simulink model "C4_closedLoopPositionPD"  (Simulink 10.2)
settings: Solver=ode4  StartTime=0.0  StopTime=1  FixedStep=T_s  RelTol=1e-3
undefined symbols (not defined in the file): b_eq, beta_p, beta_v, g, i_rated, J_eq, k, k_d_pos, k_p_currPI, k_p_pos, L, L_l, m_l, N_adc, N_e, N_opt, R, R_sh, T_i_currPI, T_s, tau_der, tau_m_rated, theta_0, theta_ref, V_adc
libraries: simulink x1
settings Model: Creator=ioannis  LastModifiedBy=mfocchi
settings DataIOCC: SaveFormat=Dataset  SignalLoggingSaveFormat=Dataset
settings OptimizationCC: LifeSpan=auto
settings DebuggingCC: UnderspecifiedInitializationDetection=Simplified  MergeDetectMultiDrivingBlocksExec=error  FcnCallInpInsideContextMsg=error  SFUnexpectedBacktrackingDiag=error  SFNoUnconditionalDefaultTransitionDiag=error  SFExecutionAtInitializationDiag=warning
settings HardwareCC: ProdBitPerPointer=64  ProdBitPerSizeT=64  ProdBitPerPtrDiffT=64  ProdLargestAtomicFloat=Float  ProdIntDivRoundTo=Zero  ProdEndianess=LittleEndian  ProdWordSize=64  ProdHWDeviceType=Intel->x86-64 (Windows64)
settings ModelReferenceCC: PropagateSignalLabelsOutOfModel=on
settings SFSimCC: SimUseLocalCustomCode=on
settings RTWCC: RTWUseLocalCustomCode=on
settings CodeAppCC: StateflowObjectComments=off
settings GRTTargetCC: TargetLangStandard=C99 (ISO)  CombineOutputUpdateFcns=on  GRTInterface=off
settings ConfigComp: CovMetricSettings=dwe  CovSaveCumulativeToWorkspaceVar=off  CovSaveSingleToWorkspaceVar=off  CovExternalEMLEnable=on

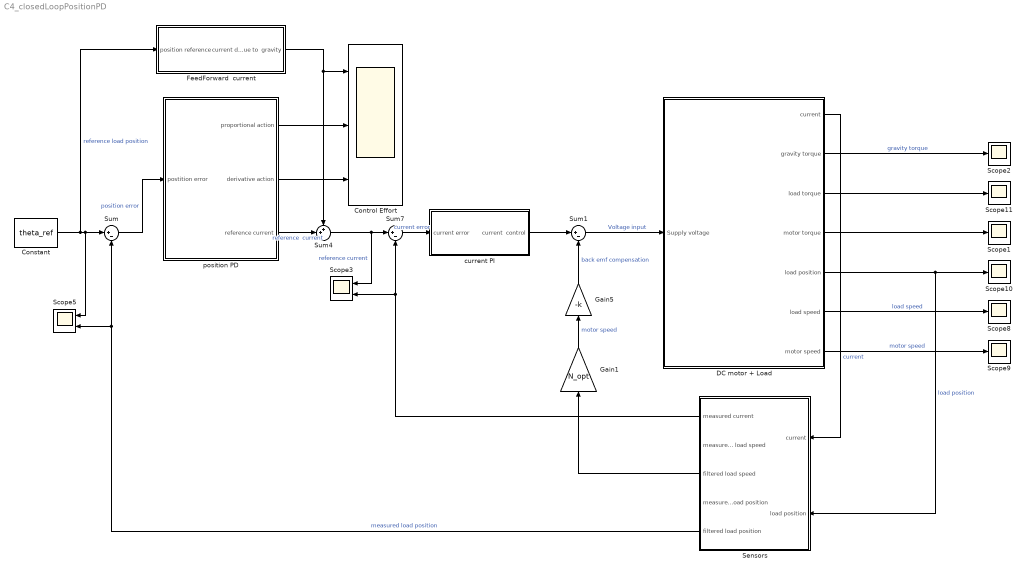
== system C4_closedLoopPositionPD ==
  Constant : Constant  Value=theta_ref
  Control Effort : Scope  NumInputPorts=3
  DC motor + Load : Subsystem
  FeedForward  current : Subsystem
  Gain1 : Gain  Gain=N_opt
  Gain5 : Gain  Gain=-k
  Scope{1..2,8..11} (6 alike) : Scope
  Scope3 : Scope  NumInputPorts=2
  Scope5 : Scope  NumInputPorts=2
  Sensors : Subsystem
  Sum : Sum  Inputs=|+-
  Sum1 : Sum  Inputs=|+-
  Sum4 : Sum  Inputs=++|
  Sum7 : Sum  Inputs=|+-
  current PI : Subsystem
  position PD : Subsystem
  wires:
  Sum7/1 -> current PI/1(current error)  "current error"
  Sum1/1 -> DC motor + Load/1(Supply voltage)  "Voltage input"
  DC motor + Load/4(motor torque) -> Scope1/1
  DC motor + Load/5(load position) -> Sensors/2(load position), Scope10/1  "load position"
  DC motor + Load/6(load speed) -> Scope8/1  "load speed"
  DC motor + Load/7(motor speed) -> Scope9/1  "motor speed"
  DC motor + Load/2(gravity torque) -> Scope2/1  "gravity torque"
  DC motor + Load/3(load torque) -> Scope11/1
  Gain1/1 -> Gain5/1  "motor speed"
  DC motor + Load/1(current) -> Sensors/1(current)  "current"
  Sensors/3(filtered load speed) -> Gain1/1
  Gain5/1 -> Sum1/2  "back emf compensation"
  Sensors/1(measured current) -> Scope3/2, Sum7/2
  Sum/1 -> position PD/1(postition error)  "position error"
  Sensors/5(filtered load position) -> Scope5/2, Sum/2  "measured load position"
  Constant/1 -> FeedForward  current/1(position reference), Scope5/1, Sum/1  "reference load position"
  current PI/1(current  control) -> Sum1/1
  Sum4/1 -> Scope3/1, Sum7/1  "reference current"
  position PD/3(reference current) -> Sum4/2  "reference  current"
  position PD/2(derivative action) -> Control Effort/3
  position PD/1(proportional action) -> Control Effort/2
  FeedForward  current/1(current due to  gravity) -> Sum4/1, Control Effort/1

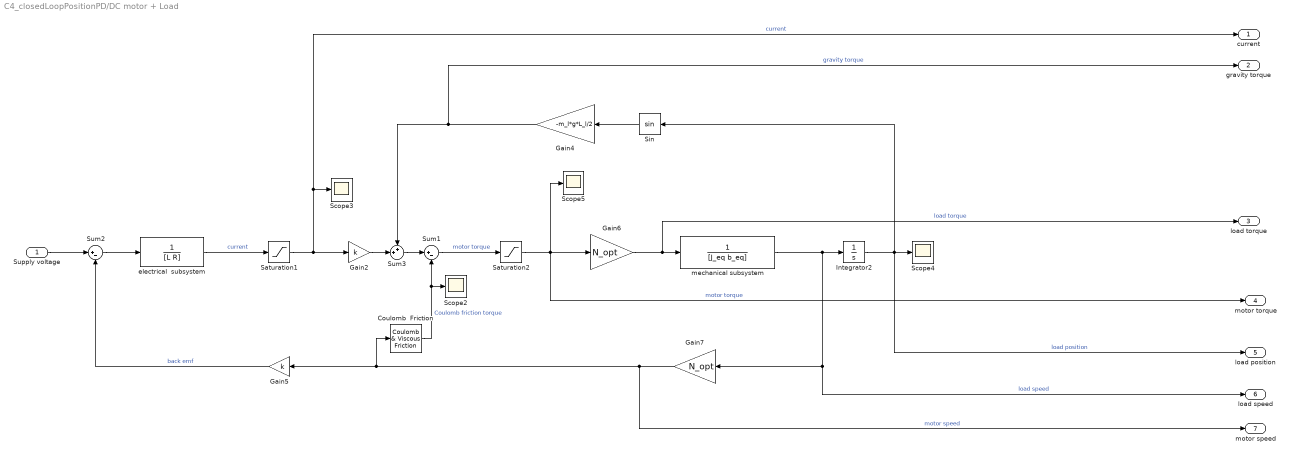
== system C4_closedLoopPositionPD/DC motor + Load ==
  Supply voltage : Inport
  Coulomb  Friction : simulink/Discontinuities/Coulomb & Viscous Friction  offset=tau_c  gain=0
  Gain2 : Gain  Gain=k
  Gain4 : Gain  Gain=-m_l*g*L_l/2
  Gain5 : Gain  Gain=k
  Gain6 : Gain  Gain=N_opt
  Gain7 : Gain  Gain=N_opt
  Integrator2 : Integrator  InitialCondition=theta_0
  Saturation1 : Saturate  UpperLimit=i_rated  LowerLimit=-i_rated
  Saturation2 : Saturate  UpperLimit=tau_m_rated  LowerLimit=-tau_m_rated
  Scope{2..5} (4 alike) : Scope
  Sin : Trigonometry
  Sum1 : Sum  Inputs=|+-
  Sum2 : Sum  Inputs=|+-
  Sum3 : Sum  Inputs=++|
  electrical  subsystem : TransferFcn  Denominator=[L R]
  mechanical subsystem : TransferFcn  Denominator=[J_eq b_eq]
  current : Outport
  gravity torque : Outport  Port=2
  load torque : Outport  Port=3
  motor torque : Outport  Port=4
  load position : Outport  Port=5
  load speed : Outport  Port=6
  motor speed : Outport  Port=7
  wires:
  Sum2/1 -> electrical  subsystem/1
  Saturation2/1 -> motor torque/1, Scope5/1, Gain6/1  "motor torque"
  Sum3/1 -> Sum1/1
  Sum1/1 -> Saturation2/1  "motor torque"
  Sin/1 -> Gain4/1
  Gain5/1 -> Sum2/2  "back emf"
  electrical  subsystem/1 -> Saturation1/1  "current"
  Gain2/1 -> Sum3/2
  Gain6/1 -> load torque/1, mechanical subsystem/1  "load torque"
  mechanical subsystem/1 -> Gain7/1, load speed/1, Integrator2/1  "load speed"
  Supply voltage/1 -> Sum2/1
  Integrator2/1 -> Sin/1, load position/1, Scope4/1  "load position"
  Gain4/1 -> gravity torque/1, Sum3/1  "gravity torque"
  Saturation1/1 -> current/1, Scope3/1, Gain2/1  "current"
  Gain7/1 -> motor speed/1, Coulomb  Friction/1, Gain5/1  "motor speed"
  Coulomb  Friction/1 -> Sum1/2, Scope2/1  "Coulomb friction torque"

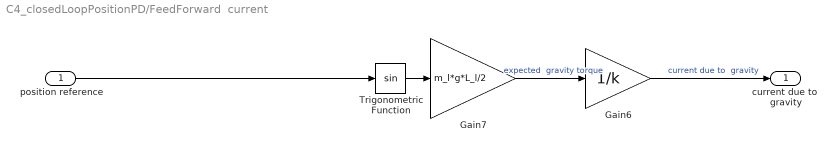
== system C4_closedLoopPositionPD/FeedForward  current ==
  position reference : Inport
  Gain6 : Gain  Gain=1/k
  Gain7 : Gain  Gain=m_l*g*L_l/2
  Trigonometric Function : Trigonometry
  current due to  gravity : Outport
  wires:
  position reference/1 -> Trigonometric Function/1
  Gain6/1 -> current due to  gravity/1  "current due to  gravity"
  Gain7/1 -> Gain6/1  "expected  gravity torque"
  Trigonometric Function/1 -> Gain7/1

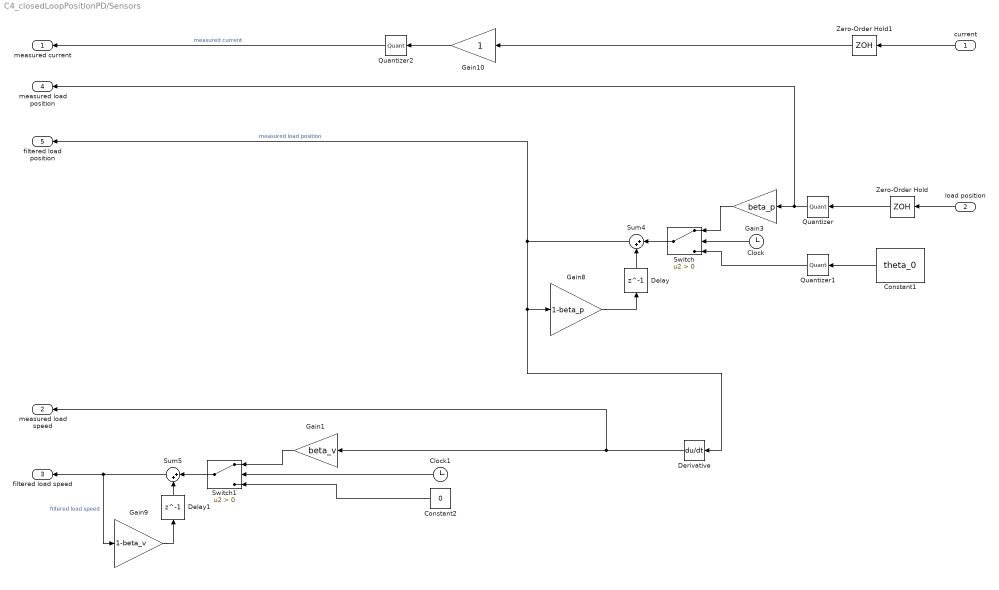
== system C4_closedLoopPositionPD/Sensors ==
  current : Inport
  load position : Inport  Port=2
  Clock : Clock
  Clock1 : Clock
  Constant1 : Constant  Value=theta_0
  Constant2 : Constant  Value=0
  Delay : Delay  DelayLength=1  InitialCondition=0
  Delay1 : Delay  DelayLength=1  InitialCondition=0
  Derivative : Derivative
  Gain1 : Gain  Gain=beta_v
  Gain10 : Gain
  Gain3 : Gain  Gain=beta_p
  Gain8 : Gain  Gain=1-beta_p
  Gain9 : Gain  Gain=1-beta_v
  Quantizer : Quantizer  QuantizationInterval=2*pi/(2^N_e)
  Quantizer1 : Quantizer  QuantizationInterval=2*pi/(2^N_e)
  Quantizer2 : Quantizer  QuantizationInterval=V_adc/R_sh/(2^N_adc)
  Sum4 : Sum  Inputs=|++
  Sum5 : Sum  Inputs=|++
  Switch : Switch  Criteria=u2 > Threshold
  Switch1 : Switch  Criteria=u2 > Threshold
  Zero-Order Hold : ZeroOrderHold  SampleTime=T_s
  Zero-Order Hold1 : ZeroOrderHold  SampleTime=T_s
  measured current : Outport
  measured load speed : Outport  Port=2
  filtered load speed : Outport  Port=3
  measured load position : Outport  Port=4
  filtered load position : Outport  Port=5
  wires:
  Gain3/1 -> Switch/1
  Switch/1 -> Sum4/1
  Quantizer/1 -> measured load position/1, Gain3/1
  Constant1/1 -> Quantizer1/1
  Delay/1 -> Sum4/2
  Quantizer1/1 -> Switch/3
  Quantizer2/1 -> measured current/1  "measured current"
  Gain10/1 -> Quantizer2/1
  Clock/1 -> Switch/2
  current/1 -> Zero-Order Hold1/1
  load position/1 -> Zero-Order Hold/1
  Sum4/1 -> filtered load position/1, Derivative/1, Gain8/1  "measured load position"
  Gain8/1 -> Delay/1
  Zero-Order Hold/1 -> Quantizer/1
  Zero-Order Hold1/1 -> Gain10/1
  Clock1/1 -> Switch1/2
  Switch1/1 -> Sum5/1
  Sum5/1 -> filtered load speed/1, Gain9/1  "filtered load speed"
  Gain1/1 -> Switch1/1
  Delay1/1 -> Sum5/2
  Gain9/1 -> Delay1/1
  Constant2/1 -> Switch1/3
  Derivative/1 -> measured load speed/1, Gain1/1

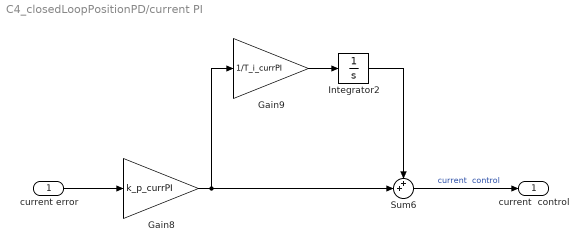
== system C4_closedLoopPositionPD/current PI ==
  current error : Inport
  Gain8 : Gain  Gain=k_p_currPI
  Gain9 : Gain  Gain=1/T_i_currPI
  Integrator2 : Integrator
  Sum6 : Sum  Inputs=++|
  current  control : Outport
  wires:
  Integrator2/1 -> Sum6/1
  Gain8/1 -> Sum6/2, Gain9/1
  current error/1 -> Gain8/1
  Sum6/1 -> current  control/1  "current  control"
  Gain9/1 -> Integrator2/1

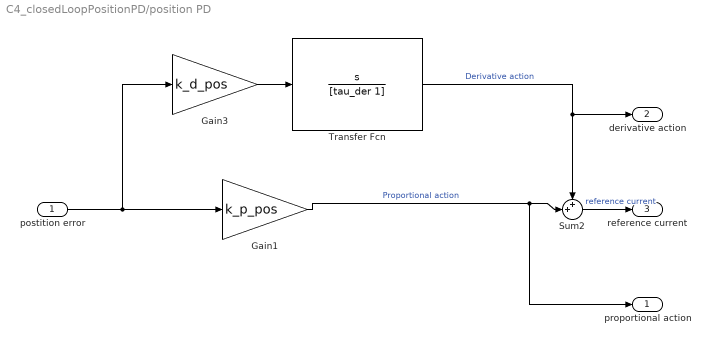
== system C4_closedLoopPositionPD/position PD ==
  postition error : Inport
  Gain1 : Gain  Gain=k_p_pos
  Gain3 : Gain  Gain=k_d_pos
  Sum2 : Sum  Inputs=++|
  Transfer Fcn : TransferFcn  Numerator=[1 0]  Denominator=[tau_der 1]
  proportional action : Outport
  derivative action : Outport  Port=2
  reference current : Outport  Port=3
  wires:
  postition error/1 -> Gain3/1, Gain1/1
  Transfer Fcn/1 -> derivative action/1, Sum2/1  "Derivative action"
  Sum2/1 -> reference current/1  "reference current"
  Gain1/1 -> proportional action/1, Sum2/2  "Proportional action"
  Gain3/1 -> Transfer Fcn/1
